simulink model "Virtual_Veh_Sim_EV3M_DLC"  (R2020a)
settings: configuration reference "Config_VarStep_Lat" (kept outside this file)
model workspace (MAT data in the model file):
  A = 159.22
  AccPwrbp = [0 0]
  AccSpdbp = [300 750]
  Aeff = 0.0314159265359
  Af = 2.46
  AfrStoich = 14.6
  AxlIxx = 62.3745166667
  AxlM = 160
  B = 1.01
  BattCapInit = 3.18
  BattCapInit_EV = 4.24
  BattChargeMax = 5.3
  BattChrgPwrMax = -60000
  BattChrgPwrMax_EV = -350000
  BattCurrMax = 300
  BattCurrMax_EV = 900
  BattDischrgPwrMax = 85000
  BattDischrgPwrMax_EV = 497000
  BattTempBp = [243.1 253.1 263.1 273.1 283.1 298.1 313.1]
  Battery : object (value not decoded)
  BrkPrsMax = 8273709
  Bx = 10
  C = 0.3618
  CapLUTBp = [0 0.01 0.02 0.03 0.04 0.05 0.06 0.07 0.08 0.09 0.1 0.11 ... (101 elements, 1x101)]
  CapSOCBp = [0 0.2 0.4 0.6 0.8 1]
  CatLightOffTime = 0
  Cd = 0.25
  ChrgLmt_bpt = [1 1 1 1 1 1 1 0.9 0.7 0.5 0]
  Cl = 0.1
  Cpm = 0.1
  Cps = 2
  CrankSpeed = 150
  Cx = 1.65
  Cz = 5565.2246438
  CzWhlAxl = 11490.971257
  DCT_Param : object (value not decoded)
  DischrgLmt_bpt = [0 0.5 0.7 0.9 1 1 1 1 1 1 1]
  Dn_Shft_Spd = [3 3 10 10 7 7 17 17 11 11 26 26 ... (20 elements, 4x5)]
  Downshift_Speeds = [9.5625 12.9375 16.3125 19.6875 23.0625 26.4375 29.8125 33.1875 36.5625 39.9375 43.3125 46.6875 ... (28 elements, 4x7)]
  Dx = 1
  ECMS_Ki = 0.1
  ECMS_Kp = 3
  ECMS_method = 1
  ECMS_s = 3.4
  Em = [2.8 3.228 3.284 3.361 3.408 3.427 3.472 3.477 3.493 3.504 3.516 3.528 ... (101 elements, 1x101)]
  EngStopStartEnable = 1
  EngStopTime : Simulink.Parameter (value not decoded)
  EngTrqCmd_0 = [0 5.91462851599 6.30130128159 6.63745773103 6.93103920513 7.1887141028 7.41614736865 7.6182009157 7.79908238179 7.96245469721 8.11151569725 8.24905488129 ... (21 elements, 1x21)]
  Ex = 0.01
  F0z = [2886 2907]
  F0zWhlAxl = 2907
  FZMAX = 6570
  FZMIN = 0
  Fc = 500
  FsbF = [-700000 -7000 -700 0 700 7000 700000]
  FsbR = [-700000 -7000 -700 0 700 7000 700000]
  FskF = [-8928.57142857 -178.571428571 0 357.142857143 535.714285714 9285.71428571]
  FskR = [-5357.14285714 -107.142857143 0 214.285714286 321.428571429 5571.42857143]
  G = [-1 0 1 2 3 4 5 6]
  G_o = 1
  Gear_Dn_bpt = [2 3 4 5 6]
  Gear_Up_bpt = [1 2 3 4 5]
  HEVEngTrq_min = 16.186104388
  Hmax = 0.25
  Iyy = 3000
  Iyy_Whl = 0.8
  J = 0.01
  J1 = 0.01
  J2 = 0.01
  Jd = 0.025
  Ji = 0.1
  Jin = 0.05
  Jin_Cltch = 0.2
  Jin_Cltch2 = 0.01
  Jout = [0.01 0.009 0.01 0.01 0.01 0.01 0.01 0.01]
  Jout_Cltch = 0.01
  Jout_Cltch2 = 0.05
  Jt = 0.1
  Jw1 = 0.01
  Jw2 = 0.01
  K_c = 10000
  Kpt = 12798
  Kz = 52451.0065793
  KzWhlAxl = 138031.612078
  LHV = 43000000
  Lhv = 42940000
  Lrel = 0.15
  Mass = 1623
  MaxTorque = [10.8721902117 76.2227873944 95.7133163788 115.203846226 134.694376076 154.184905918 173.675435766 181.839920951 181.509869828 181.17981871 180.849767971 180.519716854 ... (21 elements, 21x1)]
  N = [3.39 1 4.212 2.637 1.8 1.386 1 0.772]
  NCyl = 4
  NF = 2
  NR = 2
  N_P0 = 3
  N_P4 = 4.1
  N_idle = 750
  Ndiff = 3.32
  Ndiff_P4 = 4.1
  Ndiff_front = 5
  Ndiff_rear = 3.5
  Ndisk = 1
  Ndisks = 4
  Ngrid = 200
  Np = 2
  Np_EV = 35
  Np_FC = 1
  Ns = 72
  Ns_EV = 96
  Pabs = 101325
  Pdl_Pos_Dn_bpt = [0 0.6 0.9 1]
  Pdl_Pos_Up_bpt = [0 0.25 0.9 1]
  Pedal_Positions = [0.1 0.4 0.5 0.9]
  PenaltyFctr = 10000000
  Plimit = 60000
  Plimit_EV = 350000
  Press = 7000000
  Pstd = 101325
  RInt = [0.008846 0.006389 0.004364 0.002031 0.001443 0.0005603 0.001028 0.009319 0.006554 0.004101 0.002563 0.001825 ... (42 elements, 7x6)]
  Rair = 287
  Re = 0.327
  Reff = 0.11
  Reff_LSD = 0.2
  RegenBrkCutOff = [0 1]
  RegenBrkSpd_bpt = [2.2352 4.4704]
  Rm = 0.15
  SOCInit = 0.5
  SOCTrgt = 60
  SOC_bpt = [0 0.1 0.2 0.3 0.4 0.5 0.6 0.7 0.8 0.9 1]
  SOCmax = 80
  SOCmin = 40
  SUS : object (value not decoded)
  Sg = 0.743
  Sinj = 6.45161290323
  T = 273
  TCopy = 300
  T_eff_bp = [0 20 40 60 80 100 120 140 160 180 200]
  T_eff_bp_EV_front = [0 30 60 90 120 150 180 210 240 270 300]
  T_eff_bp_EV_rear = [0 20 40 60 80 100 120 140 160 180 200]
  T_eff_bp_P0 = [0 5.78745247607 6.36619772368 7.07355302631 7.95774715459 9.09456817668 10.6103295395 12.7323954474 15.9154943092 21.2206590789 66.6666666667]
  T_init = 298.15
  T_t = [200 200 200 200 190.9859317 143.2394488 114.591559 95.49296586 81.85111359 71.61972439 63.66197724 57.29577951 ... (14 elements, 1x14)]
  T_t_EV_front = [300 300 300 300 286.47889755 214.8591732 171.8873385 143.23944879 122.776670385 107.429586585 95.49296586 85.943669265 ... (14 elements, 1x14)]
  T_t_EV_rear = [200 200 200 200 190.9859317 143.2394488 114.591559 95.49296586 81.85111359 71.61972439 63.66197724 57.29577951 ... (14 elements, 1x14)]
  T_t_P0 = [66.6666666667 66.6666666667 66.6666666667 66.6666666667 21.2206590789 15.9154943092 12.7323954474 10.6103295395 9.09456817668 7.95774715459 7.07355302631 6.36619772368 ... (14 elements, 1x14)]
  Tc_Batt = 0.001
  Tc_DC = 0.001
  Tc_Mot = 0.02
  Temp_bpts = [313 358]
  TimeCnstECP = 0.125
  TimeCnstEGR = 0.125
  TimeCnstETC = 0.085
  TimeCnstICP = 0.125
  TimeCnstIVL = 0.125
  TimeCnstMFA = 0.125
  TimeCnstSWVA = 0.125
  TimeCnstVCR = 0.125
  TimeCnstVGT = 0.15
  TimeCnstVIRL = 0.125
  TimeCnstWGA = 0.15
  TimeStep = 0.0001
  TracPenaltyFctr = 50
  Trans : object (value not decoded)
  Trq_bpts = [25 50 75 100 150 200 250]
  Ts : Simulink.Parameter (value not decoded)
  Tstd = 293.15
  UNLOADED_RADIUS = 0.336
  Up_Shft_Spd = [5 5 12 12 9 9 19 19 13 13 28 28 ... (20 elements, 4x5)]
  Upshift_Speeds = [12.9375 16.3125 19.6875 33 26.4375 29.8125 33.1875 52.5 39.9375 43.3125 46.6875 77.25 ... (28 elements, 4x7)]
  VEH : object (value not decoded)
  VXLOW = 2
  Vd = 0.0015
  Vinit = 650
  WH : Mass (value not decoded)
  a = 3
  aMy = 0.01
  a_CG = 1.09
  afr_stoich = 14.6
  alphaMy = 0
  b : Simulink.Parameter (value not decoded)
  b1 = 100
  b1_g = 0.001
  b2 = 100
  b2_g = 0.001
  bMy = 0
  b_CG = 1.7
  b_J = 0.001
  bd = 0.001
  behavior = 0.2
  betaMy = 1
  bi = 0.001
  bin = 0.003
  bin_Cltch = 0.003
  bout = [0.003 0.003 0.003 0.003 0.003 0.003 0.003 0.003]
  bout_Cltch = 0.003
  br = 0.001
  bt = 0.001
  bw1 = 0.001
  bw2 = 0.001
  cMy = 0
  controller_type = 2
  defaultSpacing = 15
  disk_abore = 0.05
  domega_o = 0
  dt3D = 0.05
  dw = [0 10 20 40 60 80 100]
  dzdotsF = [-10 -1 -0.1 0 0.1 1 10]
  dzdotsR = [-10 -1 -0.1 0 0.1 1 10]
  dzsF = [-0.005 -0.0001 0 0.2 0.2001 0.2051]
  dzsR = [-0.005 -0.0001 0 0.2 0.2001 0.2051]
  eff = 98
  efficiency_table = [52 52 52 52 52 52 52 52 52 62 66 70 ... (154 elements, 14x11)]
  efficiency_table_EV = [85 85 85 85 85 85 85 85 85 85 85 85 ... (154 elements, 14x11)]
  efficiency_table_P0 = [52 52 52 52 52 52 52 52 52 62 66 70 ... (154 elements, 14x11)]
  egotf : object (value not decoded)
  elec_Pipe : object (value not decoded)
  elec_Radiator : object (value not decoded)
  eta = [0.95 0.95 0.95 0.95 0.95 0.95 0.95 0.95]
  eta_tbl = [0.7 0.8 0.9 0.9 0.9 0.9 0.9 0.7 0.8 0.9 0.9 0.9 ... (1232 elements, 7x11x8x2)]
  f_air = [0 0 0 0 0 0 0 0 0 0 0 0 ... (441 elements, 21x21)]
  f_co = [0 0 0 0 0 0 0 0 0 0 0 0 ... (441 elements, 21x21)]
  f_co2 = [0 0 0 0 0 0 0 0 0 0 0 0 ... (441 elements, 21x21)]
  f_cp_ld_bpt = [0 0.2 0.275 0.35 0.425 0.5 0.575 0.65 0.725 0.8 0.875 0.95 ... (16 elements, 1x16)]
  f_cp_n_bpt = [750 1053.57142857 1357.14285714 1660.71428571 1964.28571429 2267.85714286 2571.42857143 2875 3178.57142857 3482.14285714 3785.71428571 4089.28571429 ... (15 elements, 1x15)]
  f_del_sa_bpt = [0 0.75 1.5 2.25 3 3.75 4.5 5.25 6 6.75 7.5 8.25 ... (65 elements, 1x65)]
  f_ecp = [0 0 7.19012817097 15.3709456879 19.1470470057 19.0854874367 13.5819971805 0 0 0 0 0 ... (240 elements, 16x15)]
  f_eff = [499.877436556 432.508206156 399.540781628 370.894662993 347.954880181 331.11554878 319.468905906 311.408898718 305.523567029 300.961538912 297.204959405 293.79866205 ... (441 elements, 21x21)]
  f_egr_areapct_cmd = [0 3.448 6.897 10.34 13.79 17.24 20.69 24.14 27.59 31.03 34.48 37.93 ... (600 elements, 30x20)]
  f_egr_areapct_nrmlzdflow_bpt = [0 0.03448 0.06897 0.1034 0.1379 0.1724 0.2069 0.2414 0.2759 0.3103 0.3448 0.3793 ... (30 elements, 1x30)]
  f_egr_areapct_pr_bpt = [0.5 0.5263 0.5526 0.5789 0.6053 0.6316 0.6579 0.6842 0.7105 0.7368 0.7632 0.7895 ... (20 elements, 20x1)]
  f_egr_max_stdflow = [74.87 74.87 74.74 74.39 73.81 72.98 71.91 70.58 68.97 67.06 64.84 62.25 ... (20 elements, 1x20)]
  f_egr_stdflow = [0 3.743 7.487 11.23 14.97 18.72 22.46 26.2 29.95 33.69 37.43 41.18 ... (420 elements, 21x20)]
  f_egr_stdflow_egrap_bpt = [0 5 10 15 20 25 30 35 40 45 50 55 ... (21 elements, 21x1)]
  f_egr_stdflow_pr_bpt = [0.5 0.5263 0.5526 0.5789 0.6053 0.6316 0.6579 0.6842 0.7105 0.7368 0.7632 0.7895 ... (20 elements, 20x1)]
  f_egrpct_cmd = [0 0 0 0 0 0 0 0 0 0 0 0 ... (240 elements, 16x15)]
  f_egrpct_ld_bpt = [0 0.2 0.275 0.35 0.425 0.5 0.575 0.65 0.725 0.8 0.875 0.95 ... (16 elements, 1x16)]
  f_egrpct_n_bpt = [750 1054 1357 1661 1964 2268 2571 2875 3179 3482 3786 4089 ... (15 elements, 1x15)]
  f_fric_temp_bpt = [275 277 279 281 283 285 287 289 291 293 295 297 ... (46 elements, 1x46)]
  f_fric_temp_mod = [3.986 2.616 2.132 1.946 1.839 1.747 1.672 1.608 1.551 1.499 1.462 1.415 ... (46 elements, 1x46)]
  f_fuel = [0 0 0 0 0 0 0 0 0 0 0 0 ... (441 elements, 21x21)]
  f_hc = [0 0 0 0 0 0 0 0 0 0 0 0 ... (441 elements, 21x21)]
  f_icp = [0 0 1 1.09273642197 2.29409401139 3.54274371837 0.947749647567 0 0 0 0 0 ... (240 elements, 16x15)]
  f_intksys_stdflow_bpt = [0 29.67 59.34 89.01 117.8 144.1 155.7 166 175.2 183.3 190.7 197 ... (20 elements, 1x20)]
  f_intksys_stdflow_pr = [1 0.9789 0.9579 0.9368 0.9158 0.8947 0.8737 0.8526 0.8316 0.8105 0.7895 0.7684 ... (20 elements, 1x20)]
  f_lamcmd = [1 1 1 1 1 1 1 1 1 1 1 1 ... (240 elements, 16x15)]
  f_lamcmd_ld_bpt = [0 0.2 0.275 0.35 0.425 0.5 0.575 0.65 0.725 0.8 0.875 0.95 ... (16 elements, 1x16)]
  f_lamcmd_n_bpt = [750 1053.57142857 1357.14285714 1660.71428571 1964.28571429 2267.85714286 2571.42857143 2875 3178.57142857 3482.14285714 3785.71428571 4089.28571429 ... (15 elements, 1x15)]
  f_lcmd = [0 0.323404450126 0.402272754123 0.472190900601 0.545782048677 0.619112163094 0.619299299836 0.619299299836 0.619299299836 0.619299299836 0.619299299836 0.619299299836 ... (315 elements, 21x15)]
  f_lcmd_n_bpt = [750 1053.57142857 1357.14285714 1660.71428571 1964.28571429 2267.85714286 2571.42857143 2875 3178.57142857 3482.14285714 3785.71428571 4089.28571429 ... (15 elements, 1x15)]
  f_lcmd_tq_bpt = [0 15 25.2631578947 35.5263157895 45.7894736842 56.0526315789 66.3157894737 76.5789473684 86.8421052632 97.1052631579 107.368421053 117.631578947 ... (21 elements, 1x21)]
  f_m_lam = [0.94128 0.95565 0.97001 0.98437 0.99008 1.0004 0.97527 0.9549 0.92612 0.89735]
  f_m_lam_bpt = [0.65 0.7 0.75 0.8 0.85 0.9 0.95 1 1.05 1.1]
  f_m_sa = [1.0019 0.9988 0.9953 0.99173 0.98811 0.98441 0.98065 0.97682 0.97293 0.96897 0.96493 0.96083 ... (65 elements, 1x65)]
  f_mdot_air_corr = [1.02156051768 1.00597426471 0.989411677851 1.0033499089 0.984591437857 0.988509040623 1.0326198627 1.02765527362 1.0134784519 0.998280021213 0.981755128787 0.967218261288 ... (400 elements, 20x20)]
  f_mdot_air_corr_ld_bpt = [0.223381333333 0.285105122807 0.346828912281 0.408552701754 0.470276491228 0.532000280702 0.593724070175 0.655447859649 0.717171649123 0.778895438596 0.84061922807 0.902343017544 ... (20 elements, 1x20)]
  f_mdot_air_n_bpt = [750 973.6842 1197.3684 1421.0526 1644.7368 1868.4211 2092.1053 2315.7895 2539.4737 2763.1579 2986.8421 3210.5263 ... (20 elements, 1x20)]
  f_mdot_intk = [0 0 0 0 0 0 0 0 0 0 0 0 ... (400 elements, 20x20)]
  f_mdot_intk_ecp_bpt = [0 2.6316 5.2632 7.8947 10.5263 13.1579 15.7895 18.4211 21.0526 23.6842 26.3158 28.9474 ... (20 elements, 1x20)]
  f_mdot_trpd_bpt = [0 5.7895 11.5789 17.3684 23.1579 28.9474 34.7368 40.5263 46.3158 52.1053 57.8947 63.6842 ... (20 elements, 1x20)]
  f_nox = [0 0 0 0 0 0 0 0 0 0 0 0 ... (441 elements, 21x21)]
  f_nv = [0.64175366561 0.641419295169 0.640125365558 0.638690556197 0.644169906538 0.669178791311 0.731659452876 0.750078238889 0.750078238889 0.750078238889 0.750078238889 0.750078238889 ... (225 elements, 15x15)]
  f_nv_n_bpt = [750 1053.57142857 1357.14285714 1660.71428571 1964.28571429 2267.85714286 2571.42857143 2875 3178.57142857 3482.14285714 3785.71428571 4089.28571429 ... (15 elements, 1x15)]
  f_nv_prs_bpt = [31 40.6428571429 50.2857142857 59.9285714286 69.5714285714 79.2142857143 88.8571428571 98.5 108.142857143 117.785714286 127.428571429 137.071428571 ... (15 elements, 1x15)]
  f_pm = [0 0 0 0 0 0 0 0 0 0 0 0 ... (441 elements, 21x21)]
  f_sa = [9.05 9.05 16.4373253582 15.3405265461 13.6074880273 9.83352189562 3.89388784387 0 0 0 0 0 ... (240 elements, 16x15)]
  f_sa_ld_bpt = [0 0.2 0.275 0.35 0.425 0.5 0.575 0.65 0.725 0.8 0.875 0.95 ... (16 elements, 1x16)]
  f_sa_n_bpt = [750 1053.57142857 1357.14285714 1660.71428571 1964.28571429 2267.85714286 2571.42857143 2875 3178.57142857 3482.14285714 3785.71428571 4089.28571429 ... (15 elements, 1x15)]
  f_sa_opt = [35.3085 21.0105 10.3714 8.5076 7.1426 7.5656 -5.7766 -16.7061 -16.8345 -19.3546 -20.6085 -22.0872 ... (225 elements, 15x15)]
  f_startup_ect_bpt = [-40 0 20 50]
  f_startup_lambda_delta = [0.5 0.3 0.2 0]
  f_startup_lambda_delta_timecnst = [90 40 12 0]
  f_susp_axl_bp = [1 2]
  f_susp_dz_bp = [-0.325022776267 -0.315022776267 -0.305022776267 -0.205022776267 -0.105022776267 -0.00502277626717 0.0949772237328 0.194977223733 0.204977223733 0.214977223733]
  f_susp_dzdot_bp = [-3 -0.3 -0.2 -0.1 0 0.1 0.2 0.3 3]
  f_susp_fmz = [-144070.391448 -93629.24037 -75929.1118915 -20630.5828179 -15385.48216 -10140.3815021 -4895.28084414 349.819813785 -31916.3973792 18437.6709544 -83996.1993354 -33555.0482577 ... (43920 elements, 10x9x61x2x4)]
  f_susp_geom = [0 0 0 0 0 0 0 0 0 0 0 0 ... (3660 elements, 10x61x2x3)]
  f_susp_strgdelta_bp = [-0.523598775598 -0.506145483078 -0.488692190558 -0.471238898038 -0.453785605519 -0.436332312999 -0.418879020479 -0.401425727959 -0.383972435439 -0.366519142919 -0.349065850399 -0.331612557879 ... (61 elements, 1x61)]
  f_t_exh = [739.936218766 750.584766028 772.770773797 791.235245621 803.106549716 885.862998064 920.498479307 920.498479307 920.498479307 920.498479307 920.498479307 920.498479307 ... (225 elements, 15x15)]
  f_t_exh_l_bpt = [0.2 0.275 0.35 0.425 0.5 0.575 0.65 0.725 0.8 0.875 0.95 1.025 ... (15 elements, 1x15)]
  f_t_exh_n_bpt = [750 1053.57142857 1357.14285714 1660.71428571 1964.28571429 2267.85714286 2571.42857143 2875 3178.57142857 3482.14285714 3785.71428571 4089.28571429 ... (15 elements, 1x15)]
  f_tap = [0 0.9375 0.9375 0.982121188204 1.22093639741 1.5421156717 1.98870690459 2.59666257968 2.6875 2.6875 2.6875 2.6875 ... (315 elements, 21x15)]
  f_tap_ld_bpt = [0 0.2 0.268421052632 0.336842105263 0.405263157895 0.473684210526 0.542105263158 0.610526315789 0.678947368421 0.747368421053 0.815789473684 0.884210526316 ... (21 elements, 1x21)]
  f_tap_n_bpt = [750 1053.57142857 1357.14285714 1660.71428571 1964.28571429 2267.85714286 2571.42857143 2875 3178.57142857 3482.14285714 3785.71428571 4089.28571429 ... (15 elements, 1x15)]
  f_tbrake = [0 10.8721902117 10.8721902117 10.8721902117 10.8721902117 10.8721902117 10.8721902117 10.8721902117 10.8721902117 10.8721902117 10.8721902117 10.8721902117 ... (441 elements, 21x21)]
  f_tbrake_n_bpt = [0 750 973.684210526 1197.36842105 1421.05263158 1644.73684211 1868.42105263 2092.10526316 2315.78947368 2539.47368421 2763.15789474 2986.84210526 ... (21 elements, 1x21)]
  f_tbrake_t_bpt = [0 16.186104388 24.9146526824 33.6432009767 42.3717492711 51.1002975655 59.8288458599 68.5573941543 77.2859424487 86.0144907431 94.7430390375 103.471587332 ... (21 elements, 21x1)]
  f_texh = [630.359790352 638.212816583 644.85156876 656.410931683 676.180276582 706.880985433 749.880156186 804.757804763 869.00210738 938.264388175 1007.38061415 1071.70023123 ... (441 elements, 21x21)]
  f_tm_corr = [0.839360054391 0.833393271885 0.82629554201 0.818442814437 0.811524387436 0.809164184856 0.814606352881 0.826887956871 0.842304598924 0.856886829014 0.869487025783 0.880530414174 ... (400 elements, 20x20)]
  f_tm_corr_n_bpt = [750 973.6842 1197.3684 1421.0526 1644.7368 1868.4211 2092.1053 2315.7895 2539.4737 2763.1579 2986.8421 3210.5263 ... (20 elements, 1x20)]
  f_tm_corr_nd_bpt = [0.3 0.38947 0.47895 0.56842 0.65789 0.74737 0.83684 0.92632 1.0158 1.1053 1.1947 1.2842 ... (20 elements, 1x20)]
  f_tpp = [0 100]
  f_tpp_tap_bpt = [0 100]
  f_tq_fric = [4.16 4.42 4.69 4.88 4.94 4.93 4.85 4.74 4.63 4.52 4.42 4.34 ... (225 elements, 15x15)]
  f_tq_inr = [25.8508 37.8267 50.6081 62.6825 74.6026 88.9064 81.9508 76.6399 82.9886 85.0042 88.9209 92.7645 ... (225 elements, 15x15)]
  f_tq_inr_l_bpt = [0.2 0.28571 0.37143 0.45714 0.54286 0.62857 0.71429 0.8 0.88571 0.97143 1.0571 1.1429 ... (15 elements, 1x15)]
  f_tq_inr_n_bpt = [750 1053.5714 1357.1429 1660.7143 1964.2857 2267.8571 2571.4286 2875 3178.5714 3482.1429 3785.7143 4089.2857 ... (15 elements, 1x15)]
  f_tq_nl = [0 15.0012133443 26.4298333923 37.8556656512 49.2846782956 60.7113978793 72.3451969202 77.459652163 78.5324534074 78.5324534074 78.5324534074 78.5324534074 ... (256 elements, 16x16)]
  f_tq_nl_l_bpt = [0 0.2 0.275 0.35 0.425 0.5 0.575 0.65 0.725 0.8 0.875 0.95 ... (16 elements, 1x16)]
  f_tq_nl_n_bpt = [0 750 1053.57142857 1357.14285714 1660.71428571 1964.28571429 2267.85714286 2571.42857143 2875 3178.57142857 3482.14285714 3785.71428571 ... (16 elements, 1x16)]
  f_tq_pump = [7.24 5.67 3.94 2.59 1.8 1 1 1 1 1 1 1 ... (225 elements, 15x15)]
  f_twc_eff_co = [0.17 0.25 0.45 0.99 0.99 0.99 0.99]
  ... (+78 more variables)
symbols that are objects in the model workspace (value not decoded): VEH
undefined symbols (not defined in the file or in its folder): Disabled, DLCXref, DLCYref, Right, sigbuilder_block, SRE
libraries: simulink x11, vehdynlibscenariocommon x5, simulink_extras x5, vrlib x2, sim3dlib x2, vehdynlibviscommon x2, autolibshared x1, vehdynlibdriver x1, sim3dautolib x1
(part 3 of 6)

== system Virtual_Veh_Sim_EV3M_DLC/Vehicle/Drivetrain Plant Input ==
  Ctrl : Inport
  ElecFdbk : Inport  Port=2
  Env : Inport  Port=3
  Bus Selector : BusSelector  OutputSignals=PtCtrl.BrkCmd,PtCtrl.GearCmd,Steer
  Bus Selector1 : BusSelector  OutputSignals=MotTrqL,MotTrqR,MotTrqF
  Bus Selector3 : BusSelector  OutputSignals=Grade,Wind,Gnd.z.G_FL_z,Gnd.z.G_FR_z,Gnd.z.G_RL_z,Gnd.z.G_RR_z,Gnd.mu.mu_FL,Gnd.mu.mu_FR,Gnd.mu.mu_RL,Gnd.mu.mu_RR
  First Order Hold1 : FirstOrderHold  ErrorTolerance=inf
  First Order Hold2 : FirstOrderHold  ErrorTolerance=inf
  First Order Hold3 : FirstOrderHold  ErrorTolerance=inf
  Vector Concatenate : Concatenate  NumInputs=4
  Vector Concatenate1 : Concatenate  NumInputs=4
  MotTrqL : Outport  VectorParamsAs1DForOutWhenUnconnected=off
  MotTrqR : Outport  Port=2  VectorParamsAs1DForOutWhenUnconnected=off
  GearCmd : Outport  Port=3  VectorParamsAs1DForOutWhenUnconnected=off
  BrkCmd : Outport  Port=4  VectorParamsAs1DForOutWhenUnconnected=off
  Grade : Outport  Port=5  VectorParamsAs1DForOutWhenUnconnected=off
  WindVel : Outport  Port=6  VectorParamsAs1DForOutWhenUnconnected=off
  Ground : Outport  Port=7  VectorParamsAs1DForOutWhenUnconnected=off
  Friction : Outport  Port=8  VectorParamsAs1DForOutWhenUnconnected=off
  SteerAngle : Outport  Port=9  VectorParamsAs1DForOutWhenUnconnected=off
  MotTrqF : Outport  Port=10  VectorParamsAs1DForOutWhenUnconnected=off
  wires:
  Ctrl/1 -> Bus Selector/1
  ElecFdbk/1 -> Bus Selector1/1
  Bus Selector1/1 -> MotTrqL/1  "<MotTrqL>"
  Bus Selector/2 -> First Order Hold2/1  "<GearCmd>"
  Bus Selector1/2 -> MotTrqR/1  "<MotTrqR>"
  Vector Concatenate/1 -> Ground/1
  Vector Concatenate1/1 -> Friction/1
  Env/1 -> Bus Selector3/1
  Bus Selector3/4 -> Vector Concatenate/2  "<G_FR_z>"
  Bus Selector3/9 -> Vector Concatenate1/3  "<mu_RL>"
  Bus Selector3/6 -> Vector Concatenate/4  "<G_RR_z>"
  Bus Selector3/5 -> Vector Concatenate/3  "<G_RL_z>"
  Bus Selector3/3 -> Vector Concatenate/1  "<G_FL_z>"
  Bus Selector3/2 -> WindVel/1  "<Wind>"
  Bus Selector3/7 -> Vector Concatenate1/1  "<mu_FL>"
  Bus Selector3/1 -> Grade/1  "<Grade>"
  Bus Selector3/8 -> Vector Concatenate1/2  "<mu_FR>"
  Bus Selector3/10 -> Vector Concatenate1/4  "<mu_RR>"
  Bus Selector/3 -> First Order Hold3/1  "<Steer>"
  Bus Selector1/3 -> MotTrqF/1  "<MotTrqF>"
  First Order Hold1/1 -> BrkCmd/1  "BrkCmd"
  First Order Hold2/1 -> GearCmd/1  "GearCmd"
  First Order Hold3/1 -> SteerAngle/1  "SteerAngle"
  Bus Selector/1 -> First Order Hold1/1  "<BrkCmd>"

== system Virtual_Veh_Sim_EV3M_DLC/Vehicle/Electric Plant ==
  MotSpdL : Inport
  MotSpdR : Inport  Port=2
  AmbTemp : Inport  Port=3
  TorqueSplit : Inport  Port=4
  MotTrqCmdF : Inport  Port=5
  MotSpdF : Inport  Port=6
  VehSpd : Inport  Port=7
  3 Motor EV Electric Plant : Subsystem  VariantControl=1
  BattSoc : Outport
  BattPwr : Outport  Port=2
  BattCurr : Outport  Port=3
  MotTrqL : Outport  Port=4
  MotTrqR : Outport  Port=5
  MotPwrMechL : Outport  Port=6
  MotPwrElecL : Outport  Port=7
  BattV : Outport  Port=8
  MotTrqF : Outport  Port=9

== system Virtual_Veh_Sim_EV3M_DLC/Vehicle/Electric Plant Input ==
  Ctrl : Inport
  VehFdbk : Inport  Port=2
  Env : Inport  Port=3
  Bus Selector : BusSelector  OutputSignals=PtCtrl.TorqueSplit,PtCtrl.MotTrqCmdF
  Bus Selector1 : BusSelector  OutputSignals=MotSpdL,MotSpdR,MotSpdF,VehSpd
  Bus Selector2 : BusSelector  OutputSignals=Temp
  First Order Hold : FirstOrderHold  ErrorTolerance=inf
  First Order Hold1 : FirstOrderHold  ErrorTolerance=inf
  MotSpdL : Outport  VectorParamsAs1DForOutWhenUnconnected=off
  MotSpdR : Outport  Port=2  VectorParamsAs1DForOutWhenUnconnected=off
  AmbTemp : Outport  Port=3  VectorParamsAs1DForOutWhenUnconnected=off
  TorqueSplit : Outport  Port=4  VectorParamsAs1DForOutWhenUnconnected=off
  MotTrqCmdF : Outport  Port=5  VectorParamsAs1DForOutWhenUnconnected=off
  MotSpdF : Outport  Port=6  VectorParamsAs1DForOutWhenUnconnected=off
  VehSpd : Outport  Port=7  VectorParamsAs1DForOutWhenUnconnected=off
  wires:
  Ctrl/1 -> Bus Selector/1
  VehFdbk/1 -> Bus Selector1/1
  Env/1 -> Bus Selector2/1
  Bus Selector2/1 -> AmbTemp/1  "<Temp>"
  Bus Selector1/2 -> MotSpdR/1  "<MotSpdR>"
  Bus Selector1/1 -> MotSpdL/1  "<MotSpdL>"
  Bus Selector/1 -> First Order Hold/1  "<TorqueSplit>"
  Bus Selector1/3 -> MotSpdF/1  "<MotSpdF>"
  Bus Selector/2 -> First Order Hold1/1  "<MotTrqCmdF>"
  First Order Hold/1 -> TorqueSplit/1  "TorqueSplit"
  First Order Hold1/1 -> MotTrqCmdF/1  "MotTrqCmdF"
  Bus Selector1/4 -> VehSpd/1  "<VehSpd>"

== system Virtual_Veh_Sim_EV3M_DLC/Vehicle/Electric Plant Output ==
  BattSoc : Inport
  BattPwr : Inport  Port=2
  BattCurr : Inport  Port=3
  MotTrqL : Inport  Port=4
  MotTrqR : Inport  Port=5
  MotPwrMech : Inport  Port=6
  MotPwrElec : Inport  Port=7
  BattV : Inport  Port=8
  MotTrqF : Inport  Port=9
  Bus Creator1 : BusCreator  Inputs=9
  ElecFdbk : Outport  VectorParamsAs1DForOutWhenUnconnected=off
  wires:
  Bus Creator1/1 -> ElecFdbk/1  "ElecFdbk"
  BattPwr/1 -> Bus Creator1/2
  BattSoc/1 -> Bus Creator1/1
  BattCurr/1 -> Bus Creator1/3
  MotTrqL/1 -> Bus Creator1/4
  MotTrqR/1 -> Bus Creator1/5
  MotPwrMech/1 -> Bus Creator1/6
  MotPwrElec/1 -> Bus Creator1/7
  BattV/1 -> Bus Creator1/8
  MotTrqF/1 -> Bus Creator1/9

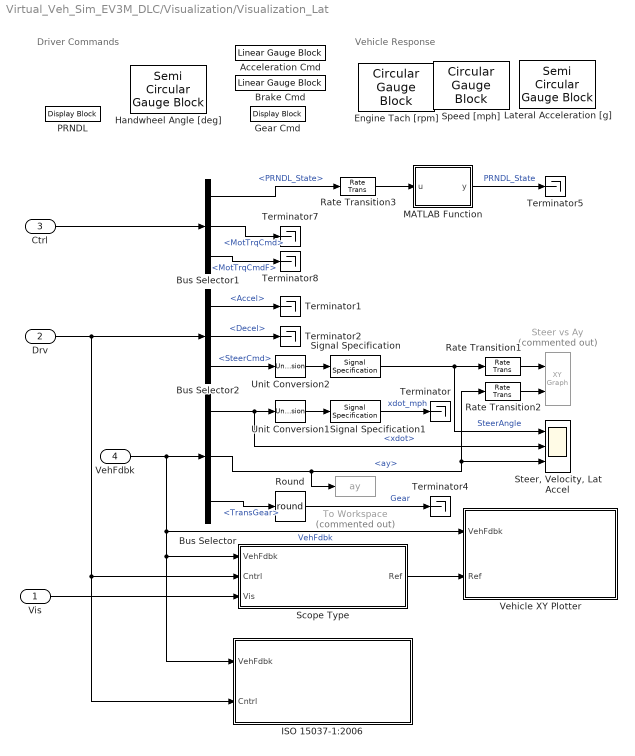
== system Virtual_Veh_Sim_EV3M_DLC/Visualization/Visualization_Lat ==
  note: Vehicle Response
  note: Driver Commands
  Vis : Inport
  Drv : Inport  Port=2
  Ctrl : Inport  Port=3
  VehFdbk : Inport  Port=4
  Acceleration Cmd : LinearGaugeBlock  LabelPosition=Hide  ScaleMax=1  TickInterval=0.20000000000000001
  Brake Cmd : LinearGaugeBlock  LabelPosition=Hide  ScaleMax=1  TickInterval=0.20000000000000001
  Bus Selector : BusSelector  OutputSignals=Veh.Body.xdot,Veh.Body.ay,Veh.TransGear
  Bus Selector1 : BusSelector  OutputSignals=PtCtrl.PRNDL_State,PtCtrl.MotTrqCmd,PtCtrl.MotTrqCmdF
  Bus Selector2 : BusSelector  OutputSignals=Accel,Decel,SteerCmd
  Engine Tach [rpm] : CircularGaugeBlock  LabelPosition=Hide  ScaleMax=8000  TickInterval=1000
  Gear Cmd : DisplayBlock  LabelPosition=Hide  Format=short  Transparency=1
  Handwheel Angle [deg] : SemiCircularGaugeBlock  LabelPosition=Hide  ScaleMin=-300  ScaleMax=300  TickInterval=60
  ISO 15037-1:2006 : Subsystem  StopFcn=|  Variant=on  VariantControlMode=Label  LabelModeActiveChoice=0  mask(ISO 15037-1:2006){Measurement=Disabled}
      | switch get_param(gcb,'Measurement')
      |     case 'Enabled'
      |        p=slproject.getCurrentProject;
      |        projectRoot=p.RootFolder;
      |        SySFolder=fullfile(projectRoot, 'System');
      |        Simulink.sdi.loadView([SySFolder filesep 'ISO15037_1_2006E.mldatx']);
      |        Simulink.sdi.view;
      | end
      mask prompts: Measurement "ISO Measurements"
      mask help: Enables display of ISO 15037-1:2006 standard measurement signals in the Simulation Data Inspector.
      mask init:
      | switch get_param(gcb,'Measurement')
      |     case 'Disabled'
      |         set_param(gcb,'OverrideUsingVariant','0')
      |     case 'Enabled'
      |        set_param(gcb,'OverrideUsingVariant','1')
      |     otherwise
      |        set_param(gcb,'OverrideUsingVariant','0')
      | end
      settings: AttributesFormatString=%<Measurement>
      mask Help: eval('vdynblkshelp(''iso15037'')');
      mask TypeOptions Measurement: Enabled | Disabled
      mask Callback Measurement:
      | switch get_param(gcb,'Measurement')
      |     case 'Disabled'
      |         set_param(gcb,'OverrideUsingVariant','0')
      |     case 'Enabled'
      |        set_param(gcb,'OverrideUsingVariant','1')
      |     otherwise
      |        set_param(gcb,'OverrideUsingVariant','0')
      | end
      mask Display: disp('ISO 15037-1:2006')
  Lateral Acceleration [g] : SemiCircularGaugeBlock  LabelPosition=Hide  ScaleMin=-1  ScaleMax=1  TickInterval=0.5
  MATLAB Function : MATLAB Function  TreatAsAtomicUnit=on
  PRNDL : DisplayBlock  LabelPosition=Hide  Format=short  Transparency=1
  Rate Transition1 : RateTransition  Deterministic=off  OutPortSampleTime=.1
  Rate Transition2 : RateTransition  Deterministic=off  OutPortSampleTime=.1
  Rate Transition3 : RateTransition  Deterministic=off  OutPortSampleTime=.1
  Round : Rounding  Operator=round
  Scope Type : Subsystem  Variant=on  VariantControlMode=Label  VariantControl=Variant1  LabelModeActiveChoice=1
  Signal Specification : SignalSpecification  Unit=deg
  Signal Specification1 : SignalSpecification  Unit=mph
  Speed [mph] : CircularGaugeBlock  LabelPosition=Hide  TickInterval=10
  Steer vs Ay : simulink/Sinks/XY Graph  Commented=on  xmin=-300  xmax=300  ymin=-1.5  ymax=1.5  st=.1
  "Steer, Velocity, Lat Accel" : Scope  NumInputPorts=3
  Terminator{,1..2,4..5,7..8} (7 alike) : Terminator
  To Workspace : ToWorkspace  Commented=on  VariableName=ay  SaveFormat=Timeseries  SampleTime=-1
  Unit Conversion1 : UnitConversion
  Unit Conversion2 : UnitConversion
  Vehicle XY Plotter : Subsystem  Variant=on  VariantControlMode=Label  VariantControl=Variant1  LabelModeActiveChoice=1
  wires:
  Signal Specification/1 -> Rate Transition1/1, "Steer, Velocity, Lat Accel"/1  "SteerAngle"
  Bus Selector/2 -> Rate Transition2/1, "Steer, Velocity, Lat Accel"/3, To Workspace/1  "<ay>"
  Bus Selector/1 -> "Steer, Velocity, Lat Accel"/2, Unit Conversion1/1  "<xdot>"
  Unit Conversion2/1 -> Signal Specification/1
  Unit Conversion1/1 -> Signal Specification1/1
  Signal Specification1/1 -> Terminator/1  "xdot_mph"
  Bus Selector2/3 -> Unit Conversion2/1  "<SteerCmd>"
  Rate Transition1/1 -> Steer vs Ay/1
  Rate Transition2/1 -> Steer vs Ay/2
  Bus Selector2/1 -> Terminator1/1  "<Accel>"
  Bus Selector2/2 -> Terminator2/1  "<Decel>"
  VehFdbk/1 -> ISO 15037-1:2006/1(VehFdbk), Scope Type/1("VehFdbk "), Vehicle XY Plotter/1("VehFdbk "), Bus Selector/1  "VehFdbk"
  Drv/1 -> ISO 15037-1:2006/2(Cntrl), Scope Type/2(Cntrl), Bus Selector2/1
  Vis/1 -> Scope Type/3("Vis ")
  Scope Type/1(" Ref") -> Vehicle XY Plotter/2("Ref ")
  Bus Selector/3 -> Round/1  "<TransGear>"
  Ctrl/1 -> Bus Selector1/1
  Bus Selector1/1 -> Rate Transition3/1  "<PRNDL_State>"
  MATLAB Function/1(y) -> Terminator5/1  "PRNDL_State"
  Round/1 -> Terminator4/1  "Gear"
  Rate Transition3/1 -> MATLAB Function/1(u)
  Bus Selector1/2 -> Terminator7/1  "<MotTrqCmd>"
  Bus Selector1/3 -> Terminator8/1  "<MotTrqCmdF>"

== system Virtual_Veh_Sim_EV3M_DLC/Controllers/Powertrain Control Module (PCM)/Powertrain Control Module (PCM) ==
  "AccelPdl " : Inport
  "DecelPdl " : Inport  Port=2
  "VehSpdFdbk " : Inport  Port=3
  "BattSoc " : Inport  Port=4
  "BattPwr " : Inport  Port=5
  "MotSpd " : Inport  Port=6
  "Chrg " : Inport  Port=7
  "BattV " : Inport  Port=8
  "TransGear " : Inport  Port=9
  MotSpdF : Inport  Port=10
  PRNDL_State : Inport  Port=11
  EV Control Module - Optimal : ModelReference  ModelNameDialog=EV_Optimal_Controller_r3.slx  SimulationMode=Normal  VariantControl=2  ModelReferenceVersion=1.4458
  " MotTrqCmd" : Outport  VectorParamsAs1DForOutWhenUnconnected=off
  " BrkCmd" : Outport  Port=2  VectorParamsAs1DForOutWhenUnconnected=off
  " WhlTrqCmd" : Outport  Port=3  VectorParamsAs1DForOutWhenUnconnected=off
  " MotTrqCmdF" : Outport  Port=4  VectorParamsAs1DForOutWhenUnconnected=off

== system Virtual_Veh_Sim_EV3M_DLC/Controllers/Powertrain Control Module (PCM)/Torque Vectoring Control ==
  MotTrqCmd : Inport
  r : Inport  Port=2
  xdot : Inport  Port=3
  WhlAng : Inport  Port=4
  MotSpdL : Inport  Port=5
  Steer : Inport  Port=6
  Brake : Inport  Port=7
  Constant Torque Split : ModelReference  ModelNameDialog=Constant_Torque_Split.slx  SimulationMode=Normal  VariantControl=0  ModelReferenceVersion=1.11
  No Torque Split : ModelReference  ModelNameDialog=No_Torque_Split.slx  SimulationMode=Normal  VariantControl=2  ModelReferenceVersion=1.10
  Torque Vectoring : ModelReference  ModelNameDialog=Torque_Vectoring.slx  SimulationMode=Normal  VariantControl=1  ModelReferenceVersion=1.25
  TQ_Split : Outport  VectorParamsAs1DForOutWhenUnconnected=off

== system Virtual_Veh_Sim_EV3M_DLC/Controllers/Powertrain Control Module (PCM)/Transmission Control Module (TCM) ==
  VehSpd : Inport
  AccelPdl : Inport  Port=2
  DecelPdl : Inport  Port=3
  PRNDL_forward : Inport  Port=4
  PRNDL_back : Inport  Port=5
  ManualShift : Inport  Port=6
  DownshiftReq : Inport  Port=7
  UpshiftReq : Inport  Port=8
  NoTCM : ModelReference  ModelNameDialog=NoTCM.slx  SimulationMode=Normal  VariantControl=2  ModelReferenceVersion=1.76
  Transmission Control Module (TCM) : ModelReference  ModelNameDialog=TransmissionController.slx  SimulationMode=Normal  VariantControl=0  ModelReferenceVersion=1.76
  GearCmd : Outport
  PRNDL_State : Outport  Port=2

== system Virtual_Veh_Sim_EV3M_DLC/Driver/Lateral Ref + DRV/Driver Commands ==
  VehRef : Inport
  VehFdbk : Inport  Port=2
  AccelGround : Ground
  BrakeGround : Ground
  Driver Commands : Subsystem  Variant=on  VariantControlMode=Label  VariantControl=Variant1  LabelModeActiveChoice=1  AllowZeroVariantControls=on
  GearGround : Ground
  SteerGround : Ground
  Driver : Outport  VectorParamsAs1DForOutWhenUnconnected=off
  wires:
  VehRef/1 -> Driver Commands/1(VehRef)
  VehFdbk/1 -> Driver Commands/2(VehFdbk)
  Driver Commands/1(" Driver") -> Driver/1
  SteerGround/1 -> Driver Commands/3(SteerCmd)
  AccelGround/1 -> Driver Commands/4(Accel)
  BrakeGround/1 -> Driver Commands/5(Brake)
  GearGround/1 -> Driver Commands/6(Gear)

== system Virtual_Veh_Sim_EV3M_DLC/Driver/Lateral Ref + DRV/Reference Generator ==
  "VehFdbk " : Inport
  3D Engine : Subsystem  Variant=on  VariantControlMode=Label  LabelModeActiveChoice=0  mask(3D Engine){engine3D=Disabled, SceneDesc=Double lane change, dt3D=dt3D, defaultPos=User-specified, X_o=X_o, Y_o=Y_o, Z_o=Z_o, phi_o=phi_o, theta_o=theta_o, psi_o=psi_o}
      mask prompts: engine3D "3D Engine"; SceneDesc "Scene:"; dt3D "Engine frame rate, dt3D [s]:"; X_o "Initial longitudinal position, X_o [m]:"; Y_o "Initial lateral position, Y_o [m]:"; Z_o "Initial vertical position, Z_o [m]:"; phi_o "Initial roll angle, phi_o [rad]:"; theta_o "Initial pitch angle, theta_o [rad]:"; psi_o "Initial yaw angle, psi_o [rad]:"
      mask help: This subsystem contains the interface blocks which permit the display of the vehicle in the 3D virtual environment. Enable it to view the simulation progress, disable it to inhibit the display.
      mask init:
      | switch get_param(gcb,'engine3D')
      |     case 'Disabled'
      |         set_param(gcb,'OverrideUsingVariant','0')
      |         try
      |             set_param([bdroot '/Environment/Ground Feedback'],'OverrideUsingVariant','0')
      |         catch
      |             disp('Warning: No ground feedback sensor not set')
      |         end
      |     case 'Enabled'
      |         set_param(gcb,'OverrideUsingVariant','1')
      |         try
      |             set_param([bdroot '/Environment/Ground Feedback'],'OverrideUsingVariant','1')
      |         catch
      |             disp('Warning: No ground feedback sensor not set')
      |         end
      |     otherwise
      |         set_param(gcb,'OverrideUsingVariant','0')
      | end
      settings: AttributesFormatString=|
      | %<SceneDesc>
      | %<engine3D>
      mask Help: eval('vdynblkshelp(''vdynblks3dengine'')');
      mask TypeOptions engine3D: Enabled | Disabled
      mask Callback engine3D:
      | switch get_param(gcb,'engine3D')
      |     case 'Disabled'
      |         set_param(gcb,'OverrideUsingVariant','0')
      |     case 'Enabled'
      |        set_param(gcb,'OverrideUsingVariant','1')
      |     otherwise
      |        set_param(gcb,'OverrideUsingVariant','0')
      | end
      mask TypeOptions SceneDesc: 3D Engine/Simulation 3D Scene Configuration/SceneDesc
      mask Callback SceneDesc: [~] = vdynblks3Dsceneconfig(gcb);
      mask TypeOptions defaultPos: Recommended for scene | User-specified
      mask DialogControl engineConfig Prompt: 3D Engine Settings
      mask DialogControl posSetup Prompt: Initial vehicle position
      mask DialogControl posSetupDesc Prompt: To use these initial vehicle positions, first Apply the initial values and then click Update the model workspaces with the initial values.
      mask DialogControl setModelPos Prompt: Update model workspaces with initial values
      mask DialogControl setModelPos Callback: [~] = vdynblksmdlWSconfig(gcb);
      mask Display: disp('3D Engine')
  Reference Generator : Subsystem  Variant=on  VariantControlMode=Label  VariantControl=Variant1  LabelModeActiveChoice=0
  " Vis" : Outport  VectorParamsAs1DForOutWhenUnconnected=off
  " Ref" : Outport  Port=2  VectorParamsAs1DForOutWhenUnconnected=off
  " Fdbk" : Outport  Port=3  VectorParamsAs1DForOutWhenUnconnected=off
  wires:
  "VehFdbk "/1 -> 3D Engine/1(VehFdbk), Reference Generator/1("VehFdbk ")
  Reference Generator/1(" Vis") -> " Vis"/1
  Reference Generator/2(" Ref") -> " Ref"/1
  Reference Generator/3(" Fdbk") -> " Fdbk"/1

== system Virtual_Veh_Sim_EV3M_DLC/Environment/Ground Feedback/3D Engine ==
  Friction : Inport
  Bus Creator : BusCreator  Inputs=4
  Bus Creator2 : BusCreator  Inputs=4
  Bus Creator3 : BusCreator  Inputs=2
  Bus Selector : BusSelector  OutputSignals=HitLoc
  Data Type Conversion : DataTypeConversion
  Demux : Demux
  Demux1 : Demux
  Passenger Vehicle Ray Trace Set : sim3dlib/Vehicle Terrain Sensor  ActorTag=SimulinkVehicle1  VehExtEn=Constant  TireRadiiExt=Constant  VehCntrLngthVal=0  TireRadiiVal=0  VehRayLngth=10  LfRayLngth=20  RfRayLngth=20  LrRayLngth=20  RrRayLngth=20  VehRayOffset=0  LfRayOffset=-1  RfRayOffset=-1  LrRayOffset=-1  RrRayOffset=-1  VehEn=on  LfEn=on  RfEn=on  LrEn=on  RrEn=on  DbgEn=off  Ts=.03  aMode=2
      settings: SourceProductBaseCode=DR,VE
  Rate Transition : RateTransition
  Reshape10 : Reshape  OutputDimensionality=Row vector (2-D)
  Selector1 : Selector  InputPortWidth=5  IndexOptions=Index vector (dialog)  Indices=[2:5]  OutputSizes=1
  Signal Specification : SignalSpecification  Unit=m
  Signal Specification1 : SignalSpecification  Unit=1
  Terminator1 : Terminator
  Terminator2 : Terminator
  Zend Select : Selector  NumberOfDimensions=2  InputPortWidth=3  IndexOptions=Select all,Index vector (dialog)  Indices=[1 3],3  OutputSizes=1,1
  Ground : Outport  VectorParamsAs1DForOutWhenUnconnected=off
  wires:
  Selector1/1 -> Rate Transition/1
  Zend Select/1 -> Reshape10/1
  Bus Selector/1 -> Zend Select/1  "<HitLoc>"
  Passenger Vehicle Ray Trace Set/2 -> Terminator1/1
  Passenger Vehicle Ray Trace Set/3 -> Terminator2/1
  Reshape10/1 -> Selector1/1
  Passenger Vehicle Ray Trace Set/1 -> Bus Selector/1
  Rate Transition/1 -> Data Type Conversion/1
  Demux/2 -> Bus Creator/2  "G_FR_z"
  Demux/1 -> Bus Creator/1  "G_FL_z"
  Demux/4 -> Bus Creator/4  "G_RR_z"
  Demux/3 -> Bus Creator/3  "G_RL_z"
  Signal Specification/1 -> Demux/1
  Signal Specification1/1 -> Demux1/1
  Demux1/1 -> Bus Creator2/1  "mu_FL"
  Bus Creator/1 -> Bus Creator3/1  "z"
  Demux1/3 -> Bus Creator2/3  "mu_RL"
  Demux1/4 -> Bus Creator2/4  "mu_RR"
  Demux1/2 -> Bus Creator2/2  "mu_FR"
  Bus Creator2/1 -> Bus Creator3/2  "mu"
  Bus Creator3/1 -> Ground/1
  Friction/1 -> Signal Specification1/1
  Data Type Conversion/1 -> Signal Specification/1

== system Virtual_Veh_Sim_EV3M_DLC/Environment/Ground Feedback/Constant ==
  Friction : Inport
  Bus Creator : BusCreator  Inputs=4
  Bus Creator2 : BusCreator  Inputs=4
  Bus Creator3 : BusCreator  Inputs=2
  Constant1 : Constant  Value=zeros(4,1)
  Demux : Demux
  Demux1 : Demux
  Signal Specification : SignalSpecification  Unit=m
  Signal Specification1 : SignalSpecification  Unit=1
  Ground : Outport  VectorParamsAs1DForOutWhenUnconnected=off
  wires:
  Constant1/1 -> Signal Specification/1
  Signal Specification/1 -> Demux/1
  Demux/4 -> Bus Creator/4  "G_RR_z"
  Demux/1 -> Bus Creator/1  "G_FL_z"
  Demux/3 -> Bus Creator/3  "G_RL_z"
  Demux/2 -> Bus Creator/2  "G_FR_z"
  Bus Creator/1 -> Bus Creator3/1  "z"
  Demux1/3 -> Bus Creator2/3  "mu_RL"
  Demux1/4 -> Bus Creator2/4  "mu_RR"
  Demux1/1 -> Bus Creator2/1  "mu_FL"
  Demux1/2 -> Bus Creator2/2  "mu_FR"
  Bus Creator2/1 -> Bus Creator3/2  "mu"
  Friction/1 -> Signal Specification1/1
  Signal Specification1/1 -> Demux1/1
  Bus Creator3/1 -> Ground/1

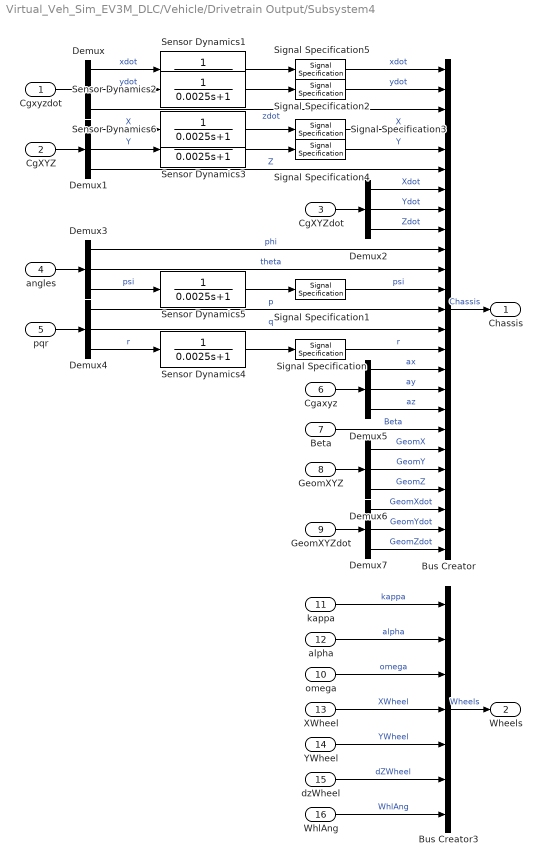
== system Virtual_Veh_Sim_EV3M_DLC/Vehicle/Drivetrain Output/Subsystem4 ==
  Cgxyzdot : Inport
  CgXYZ : Inport  Port=2
  CgXYZdot : Inport  Port=3
  angles : Inport  Port=4
  pqr : Inport  Port=5
  Cgaxyz : Inport  Port=6
  Beta : Inport  Port=7
  GeomXYZ : Inport  Port=8
  GeomXYZdot : Inport  Port=9
  omega : Inport  Port=10
  kappa : Inport  Port=11
  alpha : Inport  Port=12
  XWheel : Inport  Port=13
  YWheel : Inport  Port=14
  dzWheel : Inport  Port=15
  WhlAng : Inport  Port=16
  Bus Creator : BusCreator  Inputs=25
  Bus Creator3 : BusCreator  Inputs=7
  Demux{,1..7} (8 alike) : Demux  Outputs=3
  Sensor Dynamics{1..6} (6 alike) : TransferFcn  Denominator=[0.0025 1]
  Signal Specification : SignalSpecification  Unit=rad/s
  Signal Specification1 : SignalSpecification  Unit=rad
  Signal Specification2 : SignalSpecification  Unit=m/s
  Signal Specification3 : SignalSpecification  Unit=m
  Signal Specification4 : SignalSpecification  Unit=m
  Signal Specification5 : SignalSpecification  Unit=m/s
  Chassis : Outport  VectorParamsAs1DForOutWhenUnconnected=off
  Wheels : Outport  Port=2  VectorParamsAs1DForOutWhenUnconnected=off
  wires:
  Bus Creator/1 -> Chassis/1  "Chassis"
  omega/1 -> Bus Creator3/3  "omega"
  dzWheel/1 -> Bus Creator3/6  "dZWheel"
  kappa/1 -> Bus Creator3/1  "kappa"
  Bus Creator3/1 -> Wheels/1  "Wheels"
  YWheel/1 -> Bus Creator3/5  "YWheel"
  XWheel/1 -> Bus Creator3/4  "XWheel"
  alpha/1 -> Bus Creator3/2  "alpha"
  Cgxyzdot/1 -> Demux/1
  CgXYZ/1 -> Demux1/1
  CgXYZdot/1 -> Demux2/1
  angles/1 -> Demux3/1
  pqr/1 -> Demux4/1
  Cgaxyz/1 -> Demux5/1
  GeomXYZdot/1 -> Demux7/1
  GeomXYZ/1 -> Demux6/1
  Demux/1 -> Sensor Dynamics1/1  "xdot"
  Demux/2 -> Sensor Dynamics2/1  "ydot"
  Demux/3 -> Bus Creator/3  "zdot"
  Demux1/1 -> Sensor Dynamics6/1  "X"
  Demux1/2 -> Sensor Dynamics3/1  "Y"
  Demux1/3 -> Bus Creator/6  "Z"
  Demux2/1 -> Bus Creator/7  "Xdot"
  Demux2/2 -> Bus Creator/8  "Ydot"
  Demux2/3 -> Bus Creator/9  "Zdot"
  Demux3/1 -> Bus Creator/10  "phi"
  Demux3/2 -> Bus Creator/11  "theta"
  Demux3/3 -> Sensor Dynamics5/1  "psi"
  Demux4/1 -> Bus Creator/13  "p"
  Demux4/2 -> Bus Creator/14  "q"
  Demux4/3 -> Sensor Dynamics4/1  "r"
  Demux5/1 -> Bus Creator/16  "ax"
  Demux5/2 -> Bus Creator/17  "ay"
  Demux5/3 -> Bus Creator/18  "az"
  Beta/1 -> Bus Creator/19  "Beta"
  Demux6/1 -> Bus Creator/20  "GeomX"
  Demux6/2 -> Bus Creator/21  "GeomY"
  Demux6/3 -> Bus Creator/22  "GeomZ"
  Demux7/1 -> Bus Creator/23  "GeomXdot"
  Demux7/2 -> Bus Creator/24  "GeomYdot"
  Demux7/3 -> Bus Creator/25  "GeomZdot"
  WhlAng/1 -> Bus Creator3/7  "WhlAng"
  Sensor Dynamics1/1 -> Signal Specification5/1
  Sensor Dynamics2/1 -> Signal Specification2/1
  Sensor Dynamics3/1 -> Signal Specification4/1
  Sensor Dynamics4/1 -> Signal Specification/1
  Sensor Dynamics5/1 -> Signal Specification1/1
  Sensor Dynamics6/1 -> Signal Specification3/1
  Signal Specification/1 -> Bus Creator/15  "r"
  Signal Specification1/1 -> Bus Creator/12  "psi"
  Signal Specification2/1 -> Bus Creator/2  "ydot"
  Signal Specification3/1 -> Bus Creator/4  "X"
  Signal Specification4/1 -> Bus Creator/5  "Y"
  Signal Specification5/1 -> Bus Creator/1  "xdot"

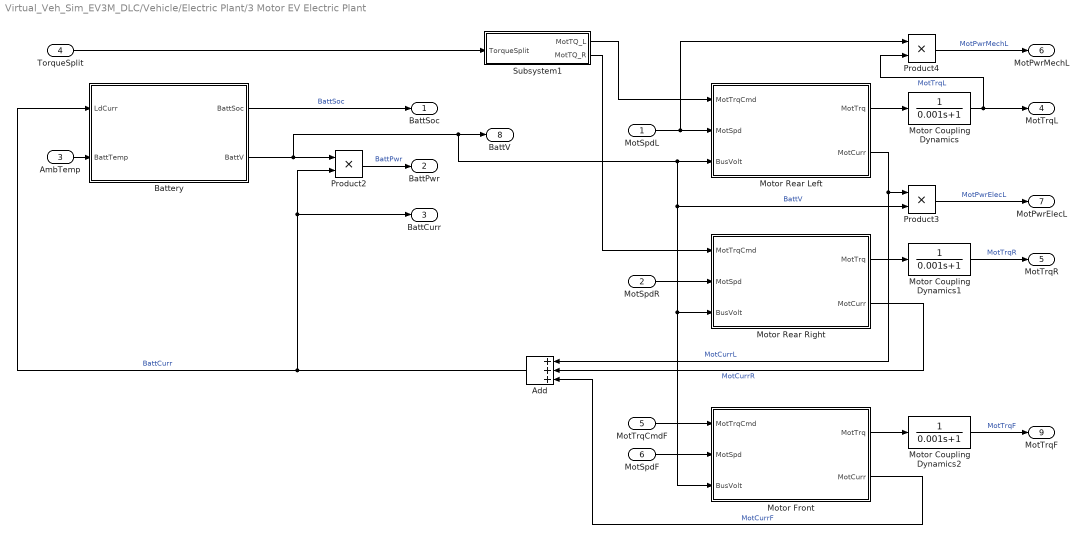
== system Virtual_Veh_Sim_EV3M_DLC/Vehicle/Electric Plant/3 Motor EV Electric Plant ==
  MotSpdL : Inport
  MotSpdR : Inport  Port=2
  AmbTemp : Inport  Port=3
  TorqueSplit : Inport  Port=4
  MotTrqCmdF : Inport  Port=5
  MotSpdF : Inport  Port=6
  Add : Sum  Inputs=+++
  Battery : Subsystem  Variant=on  VariantControlMode=Label  VariantControl=Variant1  LabelModeActiveChoice=0
  Motor Coupling Dynamics : TransferFcn  Denominator=[0.001 1]
  Motor Coupling Dynamics1 : TransferFcn  Denominator=[0.001 1]
  Motor Coupling Dynamics2 : TransferFcn  Denominator=[0.001 1]
  Motor Front : Subsystem  Variant=on  VariantControlMode=Label  LabelModeActiveChoice=0
  Motor Rear Left : Subsystem  Variant=on  VariantControlMode=Label  LabelModeActiveChoice=0
  Motor Rear Right : Subsystem  Variant=on  VariantControlMode=Label  LabelModeActiveChoice=0
  Product2 : Product
  Product3 : Product
  Product4 : Product
  Subsystem1 : Subsystem
  BattSoc : Outport  VectorParamsAs1DForOutWhenUnconnected=off
  BattPwr : Outport  Port=2  VectorParamsAs1DForOutWhenUnconnected=off
  BattCurr : Outport  Port=3  VectorParamsAs1DForOutWhenUnconnected=off
  MotTrqL : Outport  Port=4  VectorParamsAs1DForOutWhenUnconnected=off
  MotTrqR : Outport  Port=5  VectorParamsAs1DForOutWhenUnconnected=off
  MotPwrMechL : Outport  Port=6  VectorParamsAs1DForOutWhenUnconnected=off
  MotPwrElecL : Outport  Port=7  VectorParamsAs1DForOutWhenUnconnected=off
  BattV : Outport  Port=8  VectorParamsAs1DForOutWhenUnconnected=off
  MotTrqF : Outport  Port=9  VectorParamsAs1DForOutWhenUnconnected=off
  wires:
  Subsystem1/2(MotTQ_R) -> Motor Rear Right/1(MotTrqCmd)
  Subsystem1/1(MotTQ_L) -> Motor Rear Left/1(MotTrqCmd)
  TorqueSplit/1 -> Subsystem1/1(TorqueSplit)
  Motor Coupling Dynamics/1 -> MotTrqL/1, Product4/2  "MotTrqL"
  Motor Coupling Dynamics1/1 -> MotTrqR/1  "MotTrqR"
  Add/1 -> Battery/1(LdCurr), Product2/2, BattCurr/1  "BattCurr"
  MotSpdR/1 -> Motor Rear Right/2(MotSpd)
  Motor Rear Right/2(MotCurr) -> Add/2  "MotCurrR"
  Motor Rear Right/1(MotTrq) -> Motor Coupling Dynamics1/1
  Product3/1 -> MotPwrElecL/1  "MotPwrElecL"
  Product4/1 -> MotPwrMechL/1  "MotPwrMechL"
  Motor Rear Left/2(MotCurr) -> Product3/1, Add/1  "MotCurrL"
  Motor Rear Left/1(MotTrq) -> Motor Coupling Dynamics/1
  Product2/1 -> BattPwr/1  "BattPwr"
  AmbTemp/1 -> Battery/2(BattTemp)
  MotSpdL/1 -> Motor Rear Left/2(MotSpd), Product4/1
  Battery/1(BattSoc) -> BattSoc/1  "BattSoc"
  Battery/2(BattV) -> Motor Rear Left/3(BusVolt), Product3/2, Motor Front/3(BusVolt), Motor Rear Right/3(BusVolt), BattV/1, Product2/1  "BattV"
  Motor Front/1(MotTrq) -> Motor Coupling Dynamics2/1
  Motor Front/2(MotCurr) -> Add/3  "MotCurrF"
  Motor Coupling Dynamics2/1 -> MotTrqF/1  "MotTrqF"
  MotTrqCmdF/1 -> Motor Front/1(MotTrqCmd)
  MotSpdF/1 -> Motor Front/2(MotSpd)

== system Virtual_Veh_Sim_EV3M_DLC/Visualization/Visualization_Lat/ISO 15037-1:2006 ==
  VehFdbk : Inport
  Cntrl : Inport  Port=2
  Disabled : Subsystem  VariantControl=0
  Enabled : Subsystem  VariantControl=1

== system Virtual_Veh_Sim_EV3M_DLC/Visualization/Visualization_Lat/Scope Type ==
  "VehFdbk " : Inport
  Cntrl : Inport  Port=2
  "Vis " : Inport  Port=3
  DLC : Subsystem  VariantControl=1
  None : Subsystem  VariantControl=0
  XYZ : Subsystem  VariantControl=2
  " Ref" : Outport  VectorParamsAs1DForOutWhenUnconnected=off

== system Virtual_Veh_Sim_EV3M_DLC/Visualization/Visualization_Lat/Vehicle XY Plotter ==
  "VehFdbk " : Inport
  "Ref " : Inport  Port=2
  XY View : Subsystem  VariantControl=0
  XY View Ref : Subsystem  VariantControl=1

== system Virtual_Veh_Sim_EV3M_DLC/Driver/Lateral Ref + DRV/Driver Commands/Driver Commands ==
  VehRef : Inport
  VehFdbk : Inport  Port=2
  SteerCmd : Inport  Port=3
  Accel : Inport  Port=4
  Brake : Inport  Port=5
  Gear : Inport  Port=6
  Longitudinal Driver : Subsystem  VariantControl=0
  Open Loop - F310 Gamepad : Subsystem  VariantControl=4
      mask Display: image('driverlatlong.png');
  Open Loop - G29 Steering Wheel and Pedals : Subsystem  VariantControl=3
      mask Display: image('driverlatlong.png');
  Open Loop Constant Radius : Subsystem  VariantControl=2
  Predictive Driver : Subsystem  VariantControl=1
  " Driver" : Outport  VectorParamsAs1DForOutWhenUnconnected=off

== system Virtual_Veh_Sim_EV3M_DLC/Driver/Lateral Ref + DRV/Reference Generator/3D Engine ==
  note: 1) Add Subsystem or Model blocks as valid variant choices.
      | 2) You cannot connect blocks at this level. At simulation, connectivity is automatically
      | determined, based on the active variant and port name matching.
  VehFdbk : Inport
  3D Engine : Subsystem  VariantControl=1
  3D Engine Disabled : Subsystem  VariantControl=0

== system Virtual_Veh_Sim_EV3M_DLC/Driver/Lateral Ref + DRV/Reference Generator/Reference Generator ==
  "VehFdbk " : Inport
  Constant Radius : vehdynlibscenariocommon/Constant Radius  VariantControl=4  t_start=t_start  xdot_r=xdot_r  xdotUnit=mph  R=R  turnDirMask=Right  ay_max=cr_ay_max  ay_stop=off  Parameter6=2
      settings: SourceProductBaseCode=VE
  Double Lane Change : Subsystem  VariantControl=0
  Increasing Steer : Subsystem  VariantControl=1
  Open Loop - F310 Gamepad : Subsystem  VariantControl=6
  Open Loop - G29 Steering Wheel and Pedals : Subsystem  VariantControl=5
  Sine with Dwell : Subsystem  VariantControl=3
  Swept Sine : Subsystem  VariantControl=2
  " Vis" : Outport  VectorParamsAs1DForOutWhenUnconnected=off
  " Ref" : Outport  Port=2  VectorParamsAs1DForOutWhenUnconnected=off
  " Fdbk" : Outport  Port=3  VectorParamsAs1DForOutWhenUnconnected=off

== system Virtual_Veh_Sim_EV3M_DLC/Vehicle/Electric Plant/3 Motor EV Electric Plant/Battery ==
  LdCurr : Inport
  BattTemp : Inport  Port=2
  BatteryEv_3motor : ModelReference  ModelNameDialog=BattEv_3motor.slx  SimulationMode=Normal  VariantControl=0  ModelReferenceVersion=1.5656
  BattSoc : Outport  VectorParamsAs1DForOutWhenUnconnected=off
  BattV : Outport  Port=2  VectorParamsAs1DForOutWhenUnconnected=off

== system Virtual_Veh_Sim_EV3M_DLC/Vehicle/Electric Plant/3 Motor EV Electric Plant/Motor Front ==
  MotTrqCmd : Inport
  MotSpd : Inport  Port=2
  BusVolt : Inport  Port=3
  MotMapped_EV_Front : ModelReference  ModelNameDialog=MotMapped_EV_Front.slx  SimulationMode=Normal  VariantControl=0  ModelReferenceVersion=1.390
  MotTrq : Outport  VectorParamsAs1DForOutWhenUnconnected=off
  MotCurr : Outport  Port=2  VectorParamsAs1DForOutWhenUnconnected=off

== system Virtual_Veh_Sim_EV3M_DLC/Vehicle/Electric Plant/3 Motor EV Electric Plant/Motor Rear Left ==
  MotTrqCmd : Inport
  MotSpd : Inport  Port=2
  BusVolt : Inport  Port=3
  MotMapped_EV_Rear : ModelReference  ModelNameDialog=MotMapped_EV_Rear.slx  SimulationMode=Normal  VariantControl=0  ModelReferenceVersion=1.391
  MotTrq : Outport  VectorParamsAs1DForOutWhenUnconnected=off
  MotCurr : Outport  Port=2  VectorParamsAs1DForOutWhenUnconnected=off

== system Virtual_Veh_Sim_EV3M_DLC/Vehicle/Electric Plant/3 Motor EV Electric Plant/Motor Rear Right ==
  MotTrqCmd : Inport
  MotSpd : Inport  Port=2
  BusVolt : Inport  Port=3
  MotMapped_EV_Rear : ModelReference  ModelNameDialog=MotMapped_EV_Rear.slx  SimulationMode=Normal  VariantControl=0  ModelReferenceVersion=1.391
  MotTrq : Outport  VectorParamsAs1DForOutWhenUnconnected=off
  MotCurr : Outport  Port=2  VectorParamsAs1DForOutWhenUnconnected=off

== system Virtual_Veh_Sim_EV3M_DLC/Vehicle/Electric Plant/3 Motor EV Electric Plant/Subsystem1 ==
  TorqueSplit : Inport
  Demux : Demux  Outputs=2
  MotTQ_L : Outport  VectorParamsAs1DForOutWhenUnconnected=off
  MotTQ_R : Outport  Port=2  VectorParamsAs1DForOutWhenUnconnected=off
  wires:
  Demux/2 -> MotTQ_R/1
  Demux/1 -> MotTQ_L/1
  TorqueSplit/1 -> Demux/1

== system Virtual_Veh_Sim_EV3M_DLC/Visualization/Visualization_Lat/ISO 15037-1:2006/Disabled ==
  VehFdbk : Inport
  Cntrl : Inport  Port=2
  Terminator : Terminator
  Terminator1 : Terminator
  wires:
  Cntrl/1 -> Terminator/1
  VehFdbk/1 -> Terminator1/1
